simulink model "FlightDataRecorder"  (R2023b)
settings: Solver=VariableStepAuto  StartTime=0.0  StopTime=inf  RelTol=1e-3
libraries: dspindex x28, simulink x4, dspnetwork x4, etargetslib x3, aerolibconvert2 x1
(part 1 of 3)
settings Model: Creator=King  LastModifiedBy=ccInnov
settings SolverCC: AlgebraicLoopSolver=TrustRegion
settings DataIOCC: ReturnWorkspaceOutputs=off
settings OptimizationCC: BlockReduction=off
settings DebuggingCC: UnconnectedInputMsg=warning  UnconnectedOutputMsg=warning  UnconnectedLineMsg=warning  ArithmeticOperatorsInVariantConditions=warning
settings ModelReferenceCC: EnableRefExpFcnMdlSchedulingChecks=on
settings SFSimCC: SimUseLocalCustomCode=off  CustomCodeUndefinedFunction=UseInterfaceOnly
settings RTWCC: RTWUseLocalCustomCode=off
settings CodeAppCC: StateflowObjectComments=on

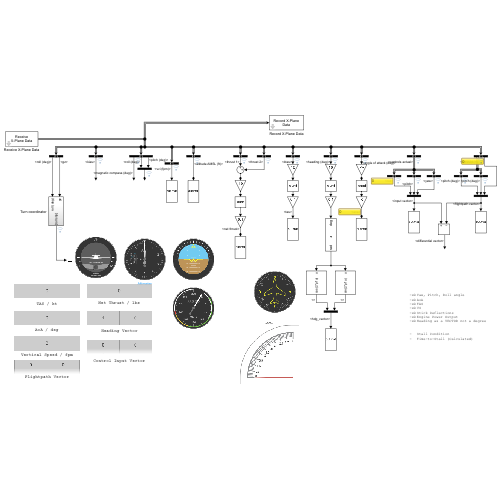
[thumbnail: Simulink's stored preview of the top-level diagram]
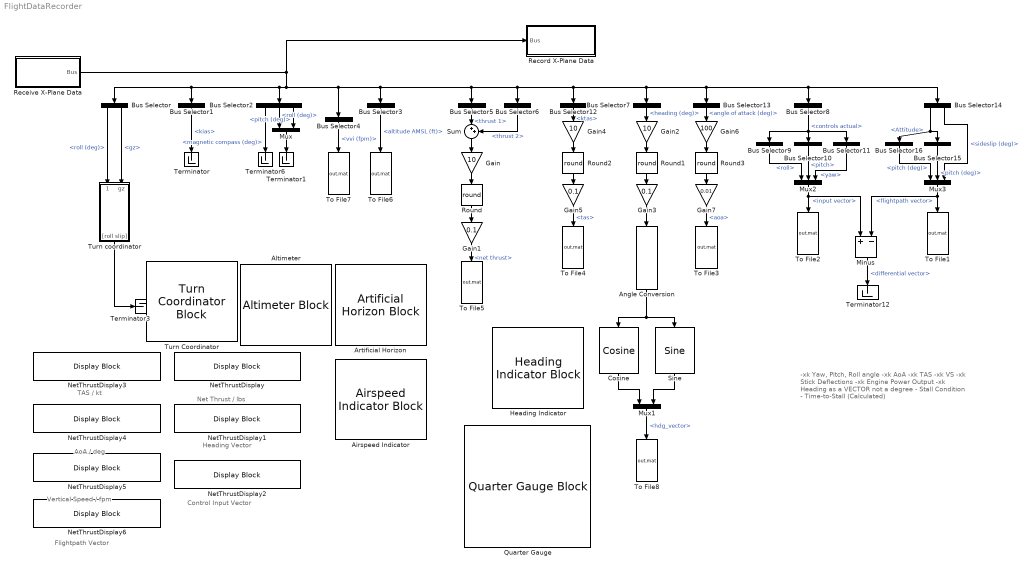
== system FlightDataRecorder ==
  note: -xk Yaw, Pitch, Roll angle
      | -xk AoA
      | -xk TAS
      | -xk VS
      | -xk Stick Deflections
      | -xk Engine Power Output
      | -xk Heading as a VECTOR not a degree
      |
      | - Stall Condition
      | - Time-to-Stall (Calculated)
  note: Net Thrust / lbs
  note: Heading Vector
  note: Control Input Vector
  note: TAS / kt
  note: AoA / deg
  note: Vertical Speed / fpm
  note: Flightpath Vector
  Airspeed Indicator : AirspeedIndicatorBlock  LabelPosition=Hide  ScaleMax=220
  Altimeter : AltimeterBlock  LabelPosition=Hide
  Angle Conversion : aerolibconvert2/Angle Conversion  IU=deg  OU=rad
  Artificial Horizon : ArtificialHorizonBlock  LabelPosition=Hide
  Bus Selector : BusSelector  OutputSignals=AHRS.Attitude.roll (deg),G-loading.gz
  Bus Selector1 : BusSelector  OutputSignals=Speeds.kias
  Bus Selector10 : BusSelector  OutputSignals=pitch
  Bus Selector11 : BusSelector  OutputSignals=yaw
  Bus Selector12 : BusSelector  OutputSignals=Speeds.ktas
  Bus Selector13 : BusSelector  OutputSignals=AHRS.Aerodynamic angles.angle of attack (deg)
  Bus Selector14 : BusSelector  OutputSignals=AHRS.Attitude,AHRS.Aerodynamic angles.sideslip (deg)
  Bus Selector15 : BusSelector  OutputSignals=pitch (deg)
  Bus Selector16 : BusSelector  OutputSignals=pitch (deg)
  Bus Selector2 : BusSelector  OutputSignals=AHRS.Compass.magnetic compass (deg),AHRS.Attitude.roll (deg),AHRS.Attitude.pitch (deg)
  Bus Selector3 : BusSelector  OutputSignals=Location.Geodetic position.altitude AMSL (ft)
  Bus Selector4 : BusSelector  OutputSignals=Speeds.vvi (fpm)
  Bus Selector5 : BusSelector  OutputSignals=Propulsion.Output.Engine thrust (lb).thrust 1
  Bus Selector6 : BusSelector  OutputSignals=Propulsion.Output.Engine thrust (lb).thrust 2
  Bus Selector7 : BusSelector  OutputSignals=AHRS.Attitude.heading (deg)
  Bus Selector8 : BusSelector  OutputSignals=Controls.Controls.controls actual
  Bus Selector9 : BusSelector  OutputSignals=roll
  Cosine : simulink/Lookup Tables/Cosine  Formula=cos(2*pi*u)  NumDataPoints=(2^5)+1  OutputWordLength=16  InternalRulePriority=Speed
  Gain : Gain  Gain=10
  Gain1 : Gain  Gain=0.1
  Gain2 : Gain  Gain=10
  Gain3 : Gain  Gain=0.1
  Gain4 : Gain  Gain=10
  Gain5 : Gain  Gain=0.1
  Gain6 : Gain  Gain=100
  Gain7 : Gain  Gain=0.01
  Heading Indicator : HeadingIndicatorBlock  LabelPosition=Hide
  Minus : Sum  Inputs=+-
  Mux : Mux  Inputs=2
  Mux1 : Mux  Inputs=2
  Mux2 : Mux  Inputs=3
  Mux3 : Mux  Inputs=3
  NetThrustDisplay{,1..6} (7 alike) : DisplayBlock  LabelPosition=Hide  Transparency=1
  Quarter Gauge : QuarterGaugeBlock  ScaleMax=3
  Receive X-Plane Data : Subsystem  mask(Receive X-Plane Data){ipaddress='127.0.0.1', sport=49000, rport=49003, Ts=0.2, p1=on, p2=on, p3=on, p4=off, p12=off, p5=off, p6=on, p7=on, p8=on, p13=off, p10=on, p9=off, p11=off, p16=off, p14=on, p15=off, p17=off, p18=off, p19=off, p20=off}
      mask prompts: ipaddress "X-Plane server IP address:"; sport "X-Plane server port:"; rport "Host data port:"; Ts "Sample time (secs)"; p1 "Time"; p2 "Speeds"; p3 "Main flight controls"; p4 "Other flight controls"; p12 "Cyclics (rotorcraft only)"; p5 "Thrust controls"; p6 "Landing gear"; p7 "AHRS data"; p8 "Engine data"; p13 "Performance data"; p10 "Forces"; p9 "Weights"; p11 "Ground effect"; p16 "Atmospheric data"; p14 "Location"; p15 "Multiplayer position data"; p17 "Power systems"; p18 "Operational systems"; p19 "NAVAID systems"; p20 "Autopilot settings"
      mask help: Configures a running instance of X-Plane to send out selected data and receives a stream of that data over UDP from X-Plane.
      mask Help: Configures a running instance of X-Plane to send out selected data and receives a stream of that data over UDP from X-Plane.
      mask DialogControl ParameterGroupVar Prompt: Network settings
      mask DialogControl Container3 Prompt: Data
      mask Display:
      | disp('Receive\nX-Plane Data')
      | %port_label('output',1,'Bus')
  Record X-Plane Data : Subsystem  mask(Record X-Plane Data){data_name='xpdata'}
      mask prompts: data_name "Data array name:"
      mask help: Records the necessary data from the data bus from the Receive X-Plane Data block for playback with the Send X-Plane Visuals block. The data store is saved to the base workspace as an array, with the X-Plane mission time for indexing the visualisation data as the first row.
      mask Help:
      | Records the necessary data from the data bus from the Receive X-Plane Data block for playback with the Send X-Plane Visuals block. The data store is saved to the base workspace as an array, with the X-Plane mission time for indexing the visualisation data as the first row.
      | 
      | The full set of data saved is:
      | 
      | > Mission time (s)
      | > Latitude (deg)
      | > Longitude (deg)
      | > Altitude MSL (m)
      | > Roll angle (deg)
      | > Pitch angle (deg)
      | > Heading (deg)
      | > Roll stick input
      | > Pitch stick input
      | > Yaw stick input
      | > Flap position
      | > Speedbrake position
      | > Gear deployment
      mask Callback data_name:
      | name = get_param(gcb,'data_name');
      | if ~strcmp(name(1),'''') || ~strcmp(name(end),'''')
      |     error('Could not update data store. Data store name must be specified as a string.',gcb);
      | else
      |     name(1) = []; name(end) = [];
      |     set_param(sprintf('%s/data store',gcb),'VariableName',name);
      | end
      mask Display:
      | disp('Record X-Plane\nData')
      | %port_label('input',1,'bus')
  Round{,1..3} (4 alike) : Rounding  Operator=round
  Sine : simulink/Lookup Tables/Sine  Formula=sin(2*pi*u)  NumDataPoints=(2^5)+1  OutputWordLength=16  InternalRulePriority=Speed
  Sum : Sum  Inputs=|++
  Terminator{,1,3,6,12} (5 alike) : Terminator
  To File1 : ToFile  Filename=out.mat  MatrixName=flightPathVector  SaveFormat=Timeseries
  To File2 : ToFile  Filename=out.mat  MatrixName=inputVector  SaveFormat=Timeseries
  To File3 : ToFile  Filename=out.mat  MatrixName=aoa  SaveFormat=Timeseries
  To File4 : ToFile  Filename=out.mat  MatrixName=tas  SaveFormat=Timeseries
  To File5 : ToFile  Filename=out.mat  MatrixName=netThrust  SaveFormat=Timeseries
  To File6 : ToFile  Filename=out.mat  MatrixName=alt  SaveFormat=Timeseries
  To File7 : ToFile  Filename=out.mat  MatrixName=vertSpeed  SaveFormat=Timeseries
  To File8 : ToFile  Filename=out.mat  MatrixName=headingVector  SaveFormat=Timeseries
  Turn Coordinator : TurnCoordinatorBlock  LabelPosition=Hide
  Turn coordinator : Subsystem
  wires:
  Receive X-Plane Data/1(Bus) -> Record X-Plane Data/1(Bus), Bus Selector/1, Bus Selector1/1, Bus Selector2/1, Bus Selector4/1, Bus Selector12/1, Bus Selector13/1, Bus Selector14/1, Bus Selector8/1, Bus Selector7/1, Bus Selector6/1, Bus Selector5/1, Bus Selector3/1
  Bus Selector1/1 -> Terminator/1  "<kias>"
  Bus Selector2/2 -> Mux/1  "<roll (deg)>"
  Bus Selector2/3 -> Mux/2  "<pitch (deg)>"
  Mux/1 -> Terminator1/1
  Bus Selector3/1 -> To File6/1  "<altitude AMSL (ft)>"
  Bus Selector/1 -> Turn coordinator/1(roll (deg))  "<roll (deg)>"
  Bus Selector/2 -> Turn coordinator/2(gz)  "<gz>"
  Turn coordinator/1("[roll slip]") -> Terminator3/1
  Bus Selector4/1 -> To File7/1  "<vvi (fpm)>"
  Bus Selector2/1 -> Terminator6/1  "<magnetic compass (deg)>"
  Bus Selector5/1 -> Sum/1  "<thrust 1>"
  Bus Selector6/1 -> Sum/2  "<thrust 2>"
  Sum/1 -> Gain/1
  Gain/1 -> Round/1
  Round/1 -> Gain1/1
  Gain1/1 -> To File5/1  "<net thrust>"
  Bus Selector7/1 -> Gain2/1  "<heading (deg)>"
  Gain2/1 -> Round1/1
  Round1/1 -> Gain3/1
  Cosine/1 -> Mux1/1
  Sine/1 -> Mux1/2
  Mux1/1 -> To File8/1  "<hdg_vector>"
  Gain3/1 -> Angle Conversion/1
  Angle Conversion/1 -> Sine/1, Cosine/1
  Bus Selector8/1 -> Bus Selector11/1, Bus Selector10/1, Bus Selector9/1  "<controls actual>"
  Bus Selector10/1 -> Mux2/2  "<pitch>"
  Bus Selector9/1 -> Mux2/1  "<roll>"
  Bus Selector11/1 -> Mux2/3  "<yaw>"
  Mux2/1 -> To File2/1, Minus/1  "<input vector>"
  Gain4/1 -> Round2/1
  Round2/1 -> Gain5/1
  Bus Selector12/1 -> Gain4/1  "<ktas>"
  Gain5/1 -> To File4/1  "<tas>"
  Round3/1 -> Gain7/1
  Gain6/1 -> Round3/1
  Gain7/1 -> To File3/1  "<aoa>"
  Bus Selector13/1 -> Gain6/1  "<angle of attack (deg)>"
  Bus Selector14/1 -> Bus Selector15/1, Bus Selector16/1  "<Attitude>"
  Bus Selector15/1 -> Mux3/2  "<pitch (deg)>"
  Bus Selector16/1 -> Mux3/1  "<pitch (deg)>"
  Bus Selector14/2 -> Mux3/3  "<sideslip (deg)>"
  Mux3/1 -> To File1/1, Minus/2  "<flightpath vector>"
  Minus/1 -> Terminator12/1  "<differential vector>"

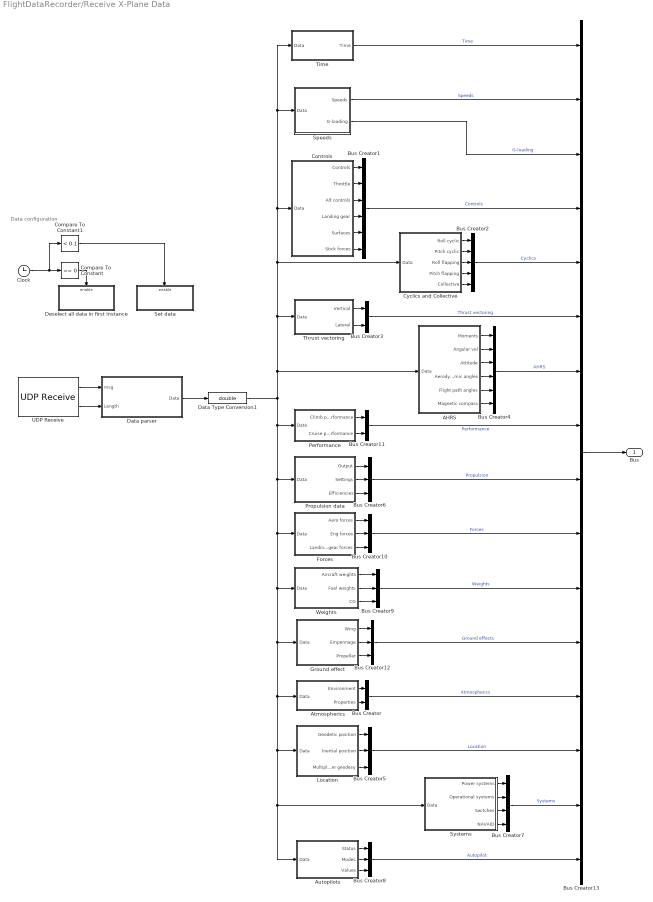
== system FlightDataRecorder/Receive X-Plane Data ==
  note: Data configuration
  AHRS : Subsystem
  Atmospherics : Subsystem
  Autopilots : Subsystem
  Bus Creator : BusCreator  Inputs=2
  Bus Creator1 : BusCreator  Inputs=6
  Bus Creator{5..6,8..10,12} (6 alike) : BusCreator  Inputs=3
  Bus Creator11 : BusCreator  Inputs=2
  Bus Creator13 : BusCreator  Inputs=16
  Bus Creator2 : BusCreator  Inputs=5
  Bus Creator3 : BusCreator  Inputs=2
  Bus Creator4 : BusCreator  Inputs=6
  Bus Creator7 : BusCreator  Inputs=4
  Clock : Clock
  Compare To Constant : simulink/Logic and Bit Operations/Compare To Constant  relop===  const=0  OutDataTypeStr=boolean
  Compare To Constant1 : simulink/Logic and Bit Operations/Compare To Constant  relop=<  const=0.1  OutDataTypeStr=boolean
  Controls : Subsystem
  Cyclics and Collective : Subsystem
  Data Type Conversion1 : DataTypeConversion  OutDataTypeStr=double  SaturateOnIntegerOverflow=off  RndMeth=Floor
  Data parser : MATLAB Function  TreatAsAtomicUnit=on
  Deselect all data in first instance : Subsystem  TreatAsAtomicUnit=on
  Forces : Subsystem
  Ground effect : Subsystem
  Location : Subsystem
  Performance : Subsystem
  Propulsion data : Subsystem
  Set data : Subsystem  TreatAsAtomicUnit=on
  Speeds : Subsystem
  Systems : Subsystem
  Thrust vectoring : Subsystem
  Time : Subsystem
  UDP Receive : dspnetwork/UDP Receive  localURL='0.0.0.0'  localPort=rport  remoteURL=ipaddress  remotePort=-1  recvBufferSize=8794  dims=4397  signalDatatype=uint8  isComplex=off  isVarSize=off  showBlockingTime=on  blockingTime=1  sampletime=Ts  blockPlatform=HOST
  Weights : Subsystem
  Bus : Outport
  wires:
  Controls/5(Surfaces) -> Bus Creator1/5
  Controls/6(Stick forces) -> Bus Creator1/6
  Controls/3(Alt controls) -> Bus Creator1/3
  Thrust vectoring/1(Vertical) -> Bus Creator3/1
  AHRS/6(Magnetic compass) -> Bus Creator4/6
  Controls/4(Landing gear) -> Bus Creator1/4
  AHRS/1(Moments) -> Bus Creator4/1
  Location/1(Geodetic position) -> Bus Creator5/1
  Systems/3(Switches) -> Bus Creator7/3
  Systems/2(Operational systems) -> Bus Creator7/2
  Weights/3(CG) -> Bus Creator9/3
  Location/2(Inertial position) -> Bus Creator5/2
  Cyclics and Collective/4(Pitch flapping) -> Bus Creator2/4
  Cyclics and Collective/2(Pitch cyclic) -> Bus Creator2/2
  Cyclics and Collective/3(Roll flapping) -> Bus Creator2/3
  AHRS/2(Angular vel) -> Bus Creator4/2
  Thrust vectoring/2(Lateral) -> Bus Creator3/2
  AHRS/3(Attitude) -> Bus Creator4/3
  AHRS/4(Aerodynamic angles) -> Bus Creator4/4
  AHRS/5(Flight path angles) -> Bus Creator4/5
  Controls/2(Throttle) -> Bus Creator1/2
  Systems/4(NAVAID) -> Bus Creator7/4
  Autopilots/2(Modes) -> Bus Creator8/2
  Autopilots/3(Values) -> Bus Creator8/3
  Location/3(Multiplayer geodesy) -> Bus Creator5/3
  Autopilots/1(Status) -> Bus Creator8/1
  Controls/1(Controls) -> Bus Creator1/1
  Weights/2(Fuel weights) -> Bus Creator9/2
  Weights/1(Aircraft weights) -> Bus Creator9/1
  Forces/1(Aero forces) -> Bus Creator10/1
  Cyclics and Collective/1(Roll cyclic) -> Bus Creator2/1
  Systems/1(Power systems) -> Bus Creator7/1
  Forces/2(Eng forces) -> Bus Creator10/2
  Forces/3(Landing gear forces) -> Bus Creator10/3
  Propulsion data/1(Output) -> Bus Creator6/1
  Ground effect/2(Empennage) -> Bus Creator12/2
  Time/1(Time) -> Bus Creator13/1  "Time"
  Propulsion data/3(Efficiencies) -> Bus Creator6/3
  Speeds/2(G-loading) -> Bus Creator13/3  "G-loading"
  Ground effect/1(Wing) -> Bus Creator12/1
  Ground effect/3(Propeller) -> Bus Creator12/3
  Propulsion data/2(Settings) -> Bus Creator6/2
  Speeds/1(Speeds) -> Bus Creator13/2  "Speeds"
  Bus Creator13/1 -> Bus/1
  Data Type Conversion1/1 -> Performance/1(Data), Forces/1(Data), Atmospherics/1(Data), Location/1(Data), Autopilots/1(Data), Systems/1(Data), Ground effect/1(Data), Weights/1(Data), Propulsion data/1(Data), AHRS/1(Data), Time/1(Data), Speeds/1(Data), Controls/1(Data), Cyclics and Collective/1(Data), Thrust vectoring/1(Data)
  Compare To Constant1/1 -> Set data/Enable
  Clock/1 -> Compare To Constant1/1, Compare To Constant/1
  Compare To Constant/1 -> Deselect all data in first instance/Enable
  UDP Receive/1 -> Data parser/1(msg)
  Data parser/1(Data) -> Data Type Conversion1/1
  UDP Receive/2 -> Data parser/2(Length)
  Cyclics and Collective/5(Collective) -> Bus Creator2/5
  Performance/1(Climb performance) -> Bus Creator11/1
  Performance/2(Cruise performance) -> Bus Creator11/2
  Atmospherics/2(Properties) -> Bus Creator/2
  Atmospherics/1(Environment) -> Bus Creator/1
  Bus Creator1/1 -> Bus Creator13/4  "Controls"
  Bus Creator2/1 -> Bus Creator13/5  "Cyclics"
  Bus Creator3/1 -> Bus Creator13/6  "Thrust vectoring"
  Bus Creator4/1 -> Bus Creator13/7  "AHRS"
  Bus Creator11/1 -> Bus Creator13/8  "Performance"
  Bus Creator6/1 -> Bus Creator13/9  "Propulsion"
  Bus Creator10/1 -> Bus Creator13/10  "Forces"
  Bus Creator9/1 -> Bus Creator13/11  "Weights"
  Bus Creator12/1 -> Bus Creator13/12  "Ground effects"
  Bus Creator/1 -> Bus Creator13/13  "Atmospherics"
  Bus Creator5/1 -> Bus Creator13/14  "Location"
  Bus Creator7/1 -> Bus Creator13/15  "Systems"
  Bus Creator8/1 -> Bus Creator13/16  "Autopilot"

== system FlightDataRecorder/Record X-Plane Data ==
  Bus : Inport
  Bus Selector : BusSelector  OutputSignals=Time.mission time,Location.Geodetic position.latitude (deg),Location.Geodetic position.longitude (deg),Location.Geodetic position.altitude AMSL (ft),AHRS.Attitude.roll (deg),AHRS.Attitude.pitch (deg),AHRS.Attitude.heading (deg),Controls.Controls.controls actual.roll,Controls.Controls.controls actual.pitch,Controls.Controls.controls actual.yaw,Controls.Controls.trim tabs.flap position,Controls.Controls.trim tabs.speedbrake actual,Controls.Landing gear.gear status  OutputAsBus=on
  data store : ToWorkspace  VariableName=xpdata  SampleTime=-1
      settings: Save2DSignal=2-D array (concatenate along first dimension)
  wires:
  Bus/1 -> Bus Selector/1
  Bus Selector/1 -> data store/1

== system FlightDataRecorder/Turn coordinator ==
  roll (deg) : Inport
  gz : Inport  Port=2
  Bias : Bias  Bias=-1  SaturateOnIntegerOverflow=off
  Gain : Gain  Gain=-1
  Mux4 : Mux  Inputs=2
  Product : Product
  Sign : Signum
  "[roll slip]" : Outport
  wires:
  Mux4/1 -> "[roll slip]"/1
  Sign/1 -> Product/1
  Bias/1 -> Product/2
  Product/1 -> Gain/1
  roll (deg)/1 -> Sign/1, Mux4/1
  gz/1 -> Bias/1
  Gain/1 -> Mux4/2

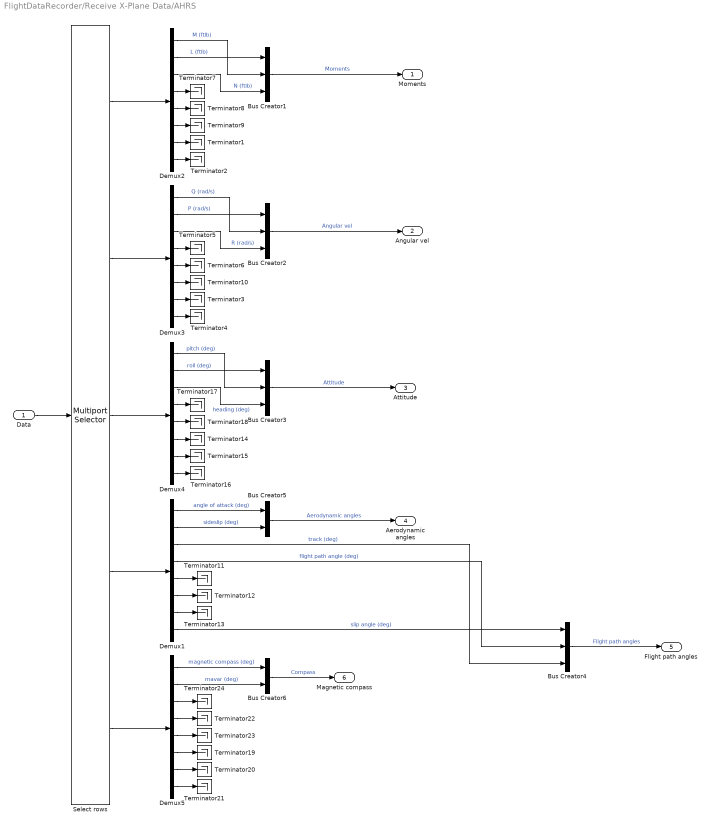
== system FlightDataRecorder/Receive X-Plane Data/AHRS ==
  Data : Inport
  Bus Creator{1..4} (4 alike) : BusCreator  Inputs=3
  Bus Creator5 : BusCreator  Inputs=2
  Bus Creator6 : BusCreator  Inputs=2
  Demux{1..5} (5 alike) : Demux  Outputs=8
  Select rows : dspindex/Multiport Selector  rowsOrCols=Rows  idxCellArray={16,17,18,19,20}  idxErrMode=Clip Index
  Terminator{1..24} (24 alike) : Terminator
  Moments : Outport
  Angular vel : Outport  Port=2
  Attitude : Outport  Port=3
  Aerodynamic angles : Outport  Port=4
  Flight path angles : Outport  Port=5
  Magnetic compass : Outport  Port=6
  wires:
  Bus Creator1/1 -> Moments/1  "Moments"
  Select rows/3 -> Demux4/1
  Select rows/2 -> Demux3/1
  Select rows/1 -> Demux2/1
  Data/1 -> Select rows/1
  Demux2/3 -> Bus Creator1/3  "N (ftlb)"
  Demux2/4 -> Terminator7/1
  Demux2/5 -> Terminator8/1
  Demux2/6 -> Terminator9/1
  Demux2/7 -> Terminator1/1
  Demux2/8 -> Terminator2/1
  Demux3/4 -> Terminator5/1
  Demux3/5 -> Terminator6/1
  Demux3/6 -> Terminator10/1
  Demux3/7 -> Terminator3/1
  Demux3/8 -> Terminator4/1
  Demux3/3 -> Bus Creator2/3  "R (rad/s)"
  Bus Creator2/1 -> Angular vel/1  "Angular vel"
  Demux4/3 -> Bus Creator3/3  "heading (deg)"
  Select rows/4 -> Demux1/1
  Demux1/1 -> Bus Creator5/1  "angle of attack (deg)"
  Demux1/2 -> Bus Creator5/2  "sideslip (deg)"
  Bus Creator3/1 -> Attitude/1  "Attitude"
  Bus Creator5/1 -> Aerodynamic angles/1  "Aerodynamic angles"
  Demux1/4 -> Bus Creator4/2  "flight path angle (deg)"
  Demux1/5 -> Terminator11/1
  Demux1/6 -> Terminator12/1
  Demux1/7 -> Terminator13/1
  Demux4/5 -> Terminator18/1
  Demux4/4 -> Terminator17/1
  Demux4/6 -> Terminator14/1
  Demux4/7 -> Terminator15/1
  Demux4/8 -> Terminator16/1
  Demux5/4 -> Terminator22/1
  Demux5/6 -> Terminator19/1
  Demux5/5 -> Terminator23/1
  Demux5/7 -> Terminator20/1
  Demux5/8 -> Terminator21/1
  Demux5/3 -> Terminator24/1
  Demux5/1 -> Bus Creator6/1  "magnetic compass (deg)"
  Demux5/2 -> Bus Creator6/2  "mavar (deg)"
  Bus Creator4/1 -> Flight path angles/1  "Flight path angles"
  Demux1/8 -> Bus Creator4/1  "slip angle (deg)"
  Demux1/3 -> Bus Creator4/3  "track (deg)"
  Bus Creator6/1 -> Magnetic compass/1  "Compass"
  Select rows/5 -> Demux5/1
  Demux4/1 -> Bus Creator3/2  "pitch (deg)"
  Demux4/2 -> Bus Creator3/1  "roll (deg)"
  Demux2/2 -> Bus Creator1/1  "L (ftlb)"
  Demux2/1 -> Bus Creator1/2  "M (ftlb)"
  Demux3/1 -> Bus Creator2/2  "Q (rad/s)"
  Demux3/2 -> Bus Creator2/1  "P (rad/s)"

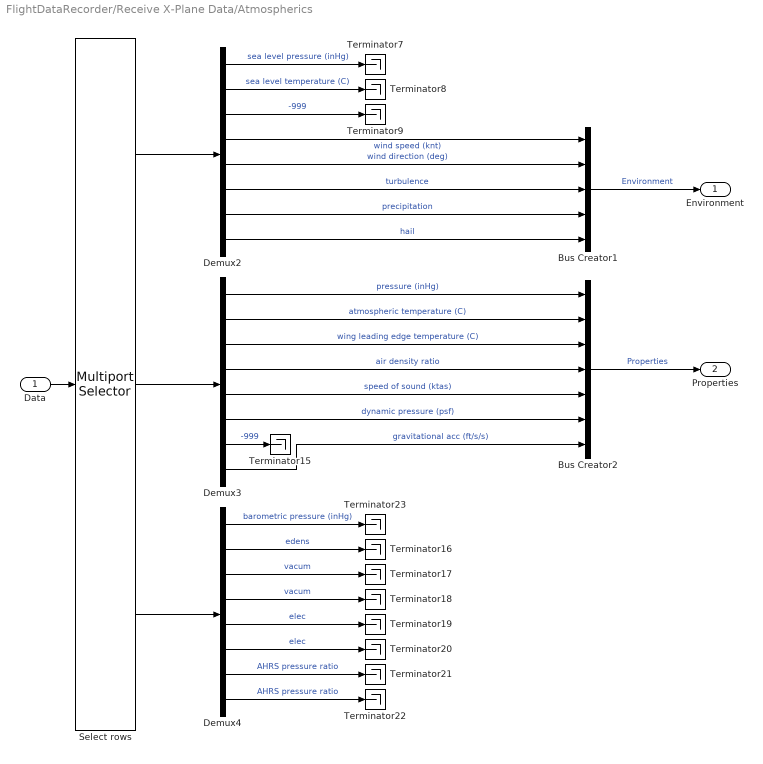
== system FlightDataRecorder/Receive X-Plane Data/Atmospherics ==
  Data : Inport
  Bus Creator1 : BusCreator  Inputs=5
  Bus Creator2 : BusCreator  Inputs=7
  Demux2 : Demux  Outputs=8
  Demux3 : Demux  Outputs=8
  Demux4 : Demux  Outputs=8
  Select rows : dspindex/Multiport Selector  rowsOrCols=Rows  idxCellArray={6,7,8}  idxErrMode=Clip Index
  Terminator{7..9,15..23} (12 alike) : Terminator
  Environment : Outport
  Properties : Outport  Port=2
  wires:
  Data/1 -> Select rows/1
  Select rows/1 -> Demux2/1
  Select rows/2 -> Demux3/1
  Select rows/3 -> Demux4/1
  Demux2/1 -> Terminator7/1  "sea level pressure (inHg)"
  Demux2/2 -> Terminator8/1  "sea level temperature (C)"
  Demux2/3 -> Terminator9/1  "-999"
  Demux3/7 -> Terminator15/1  "-999"
  Demux4/1 -> Terminator23/1  "barometric pressure (inHg)"
  Demux4/2 -> Terminator16/1  "edens"
  Demux4/3 -> Terminator17/1  "vacum"
  Demux4/4 -> Terminator18/1  "vacum"
  Demux4/5 -> Terminator19/1  "elec"
  Demux4/6 -> Terminator20/1  "elec"
  Demux4/7 -> Terminator21/1  "AHRS pressure ratio"
  Demux4/8 -> Terminator22/1  "AHRS pressure ratio"
  Bus Creator2/1 -> Properties/1  "Properties"
  Bus Creator1/1 -> Environment/1  "Environment"
  Demux2/4 -> Bus Creator1/1  "wind speed (knt)"
  Demux2/5 -> Bus Creator1/2  "wind direction (deg)"
  Demux2/6 -> Bus Creator1/3  "turbulence"
  Demux2/7 -> Bus Creator1/4  "precipitation"
  Demux2/8 -> Bus Creator1/5  "hail"
  Demux3/1 -> Bus Creator2/1  "pressure (inHg)"
  Demux3/2 -> Bus Creator2/2  "atmospheric temperature (C)"
  Demux3/3 -> Bus Creator2/3  "wing leading edge temperature (C)"
  Demux3/4 -> Bus Creator2/4  "air density ratio"
  Demux3/5 -> Bus Creator2/5  "speed of sound (ktas)"
  Demux3/6 -> Bus Creator2/6  "dynamic pressure (psf)"
  Demux3/8 -> Bus Creator2/7  "gravitational acc (ft/s/s)"

== system FlightDataRecorder/Receive X-Plane Data/Autopilots ==
  Data : Inport
  Bus Creator10 : BusCreator  Inputs=8
  Bus Creator12 : BusCreator  Inputs=6
  Bus Creator13 : BusCreator  Inputs=8
  Demux11 : Demux  Outputs=8
  Demux12 : Demux  Outputs=8
  Demux13 : Demux  Outputs=8
  Select rows1 : dspindex/Multiport Selector  rowsOrCols=Rows  idxCellArray={117,118,119}  idxErrMode=Clip Index
  Terminator17 : Terminator
  Terminator18 : Terminator
  Status : Outport
  Modes : Outport  Port=2
  Values : Outport  Port=3
  wires:
  Demux13/7 -> Bus Creator13/7  "roll sync"
  Demux13/4 -> Bus Creator13/4  "altitude dial"
  Demux13/6 -> Bus Creator13/6  "altitude use"
  Demux13/8 -> Bus Creator13/8  "pitch sync"
  Demux13/5 -> Bus Creator13/5  "vnav dial"
  Demux13/3 -> Bus Creator13/3  "vvi cmd"
  Demux13/2 -> Bus Creator13/2  "heading cmd"
  Demux13/1 -> Bus Creator13/1  "speed cmd"
  Bus Creator13/1 -> Values/1  "Autopilot values"
  Select rows1/3 -> Demux13/1
  Demux12/7 -> Terminator18/1
  Demux12/8 -> Bus Creator12/6  "sync"
  Demux12/4 -> Terminator17/1
  Demux12/6 -> Bus Creator12/5  "app"
  Demux12/5 -> Bus Creator12/4  "bac"
  Demux12/3 -> Bus Creator12/3  "altitude"
  Demux12/2 -> Bus Creator12/2  "heading"
  Demux12/1 -> Bus Creator12/1  "autothrottle"
  Bus Creator12/1 -> Modes/1  "Autopilot modes"
  Select rows1/2 -> Demux12/1
  Demux11/7 -> Bus Creator10/7  "gp enabled"
  Demux11/4 -> Bus Creator10/4  "vnav enabled"
  Demux11/6 -> Bus Creator10/6  "vnav time"
  Demux11/8 -> Bus Creator10/8  "app type"
  Demux11/5 -> Bus Creator10/5  "vnav armed"
  Demux11/3 -> Bus Creator10/3  "app armed"
  Demux11/2 -> Bus Creator10/2  "alt armed"
  Demux11/1 -> Bus Creator10/1  "nav armed"
  Bus Creator10/1 -> Status/1  "Autopilot arming"
  Select rows1/1 -> Demux11/1
  Data/1 -> Select rows1/1

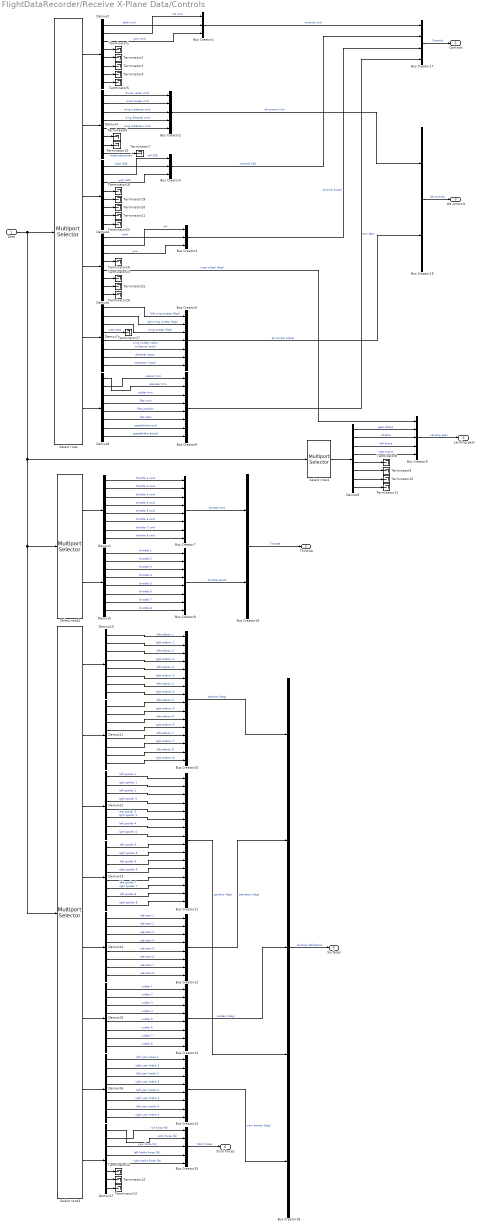
== system FlightDataRecorder/Receive X-Plane Data/Controls ==
  Data : Inport
  Bus Creator1 : BusCreator  Inputs=3
  Bus Creator10 : BusCreator  Inputs=16
  Bus Creator11 : BusCreator  Inputs=16
  Bus Creator{6..8,12..14} (6 alike) : BusCreator  Inputs=8
  Bus Creator{2,9,15,18} (4 alike) : BusCreator  Inputs=5
  Bus Creator16 : BusCreator  Inputs=2
  Bus Creator17 : BusCreator  Inputs=4
  Bus Creator19 : BusCreator  Inputs=2
  Bus Creator3 : BusCreator  Inputs=3
  Bus Creator4 : BusCreator  Inputs=3
  Bus Creator5 : BusCreator  Inputs=7
  Demux{1..17} (17 alike) : Demux  Outputs=8
  Select rows : dspindex/Multiport Selector  rowsOrCols=Rows  idxCellArray={9,10,11,12,13,14}  idxErrMode=Clip Index
  Select rows1 : dspindex/Multiport Selector  rowsOrCols=Rows  idxCellArray={15}  idxErrMode=Clip Index
  Select rows2 : dspindex/Multiport Selector  rowsOrCols=Rows  idxCellArray={26,27}  idxErrMode=Clip Index
  Select rows3 : dspindex/Multiport Selector  rowsOrCols=Rows  idxCellArray={71,72,73,74,75,76,77,78}  idxErrMode=Clip Index
  Terminator{1..23,25..26} (25 alike) : Terminator
  Controls : Outport
  Throttle : Outport  Port=2
  Alt controls : Outport  Port=3
  Landing gear : Outport  Port=4
  Surfaces : Outport  Port=5
  Stick forces : Outport  Port=6
  wires:
  Demux4/8 -> Terminator22/1
  Demux4/7 -> Terminator21/1
  Demux4/6 -> Terminator20/1
  Demux4/5 -> Terminator19/1
  Demux4/4 -> Terminator18/1
  Demux4/3 -> Bus Creator3/3  "yaw SAS"
  Demux3/7 -> Terminator15/1
  Select rows/3 -> Demux4/1
  Select rows/2 -> Demux3/1
  Select rows/1 -> Demux2/1
  Data/1 -> Select rows3/1, Select rows2/1, Select rows1/1, Select rows/1
  Demux2/4 -> Terminator1/1
  Demux2/5 -> Terminator2/1
  Demux2/6 -> Terminator3/1
  Demux2/7 -> Terminator4/1
  Demux2/8 -> Terminator5/1
  Demux2/3 -> Bus Creator1/3  "yaw cmd"
  Demux3/1 -> Bus Creator2/1  "thrust vector cmd"
  Demux3/2 -> Bus Creator2/2  "wind sweep cmd"
  Demux3/3 -> Bus Creator2/3  "wing incidence cmd"
  Demux3/4 -> Bus Creator2/4  "wing dihedral cmd"
  Demux3/5 -> Bus Creator2/5  "wing retraction cmd"
  Demux3/8 -> Terminator7/1  "water jettisoned"
  Demux3/6 -> Terminator6/1
  Select rows2/2 -> Demux5/1
  Select rows2/1 -> Demux1/1
  Bus Creator3/1 -> Bus Creator17/2  "controls SAS"
  Demux6/8 -> Terminator26/1
  Demux6/7 -> Terminator25/1
  Demux6/6 -> Terminator23/1
  Demux6/5 -> Bus Creator9/1  "nose wheel (deg)"
  Demux6/4 -> Terminator16/1
  Demux6/3 -> Bus Creator4/3  "yaw"
  Select rows/4 -> Demux6/1
  Select rows/5 -> Demux7/1
  Demux7/1 -> Bus Creator5/1  "left wing sweep (deg)"
  Demux7/3 -> Bus Creator5/3  "wing sweep (deg)"
  Demux7/4 -> Terminator17/1  "vect ratio"
  Demux7/5 -> Bus Creator5/4  "wing sweep (ratio)"
  Demux7/6 -> Bus Creator5/5  "incidence (ratio)"
  Demux7/7 -> Bus Creator5/6  "dihedral (ratio)"
  Demux7/8 -> Bus Creator5/7  "retraction (ratio)"
  Demux7/2 -> Bus Creator5/2  "right wing sweep (deg)"
  Select rows/6 -> Demux8/1
  Demux8/3 -> Bus Creator6/3  "rudder trim"
  Demux8/4 -> Bus Creator6/4  "flap cmd"
  Demux8/7 -> Bus Creator6/7  "speedbrake cmd"
  Demux8/5 -> Bus Creator6/5  "flap position"
  Demux8/6 -> Bus Creator6/6  "slat ratio"
  Demux8/8 -> Bus Creator6/8  "speedbrake actual"
  Bus Creator6/1 -> Bus Creator17/4  "trim tabs"
  Demux1/3 -> Bus Creator7/3  "throttle 3 cmd"
  Demux1/4 -> Bus Creator7/4  "throttle 4 cmd"
  Demux1/2 -> Bus Creator7/2  "throttle 2 cmd"
  Demux1/1 -> Bus Creator7/1  "throttle 1 cmd"
  Demux1/8 -> Bus Creator7/8  "throttle 8 cmd"
  Demux1/7 -> Bus Creator7/7  "throttle 7 cmd"
  Demux1/5 -> Bus Creator7/5  "throttle 5 cmd"
  Demux1/6 -> Bus Creator7/6  "throttle 6 cmd"
  Demux5/3 -> Bus Creator8/3  "throttle 3"
  Demux5/6 -> Bus Creator8/6  "throttle 6"
  Demux5/8 -> Bus Creator8/8  "throttle 8"
  Demux5/2 -> Bus Creator8/2  "throttle 2"
  Demux5/4 -> Bus Creator8/4  "throttle 4"
  Demux5/1 -> Bus Creator8/1  "throttle 1"
  Demux5/7 -> Bus Creator8/7  "throttle 7"
  Demux5/5 -> Bus Creator8/5  "throttle 5"
  Bus Creator8/1 -> Bus Creator16/2  "throttle actual"
  Bus Creator4/1 -> Bus Creator17/3  "controls actual"
  Bus Creator2/1 -> Bus Creator19/1  "alt control cmd"
  Select rows1/1 -> Demux9/1
  Demux9/5 -> Terminator8/1
  Demux9/6 -> Terminator9/1
  Demux9/7 -> Terminator10/1
  Demux9/8 -> Terminator11/1
  Demux9/1 -> Bus Creator9/2  "gear status"
  Demux9/2 -> Bus Creator9/3  "wbrake"
  Demux9/3 -> Bus Creator9/4  "left brake"
  Demux9/4 -> Bus Creator9/5  "right brake"
  Bus Creator9/1 -> Landing gear/1  "Landing gear"
  Demux10/3 -> Bus Creator10/3  "left aileron 2"
  Demux10/6 -> Bus Creator10/6  "right aileron 3"
  Demux10/8 -> Bus Creator10/8  "right aileron 4"
  Demux10/2 -> Bus Creator10/2  "right aileron 1"
  Demux10/4 -> Bus Creator10/4  "right aileron 2"
  Demux10/7 -> Bus Creator10/7  "left aileron 4"
  Demux10/5 -> Bus Creator10/5  "left aileron 3"
  Bus Creator10/1 -> Bus Creator18/1  "ailerons (deg)"
  Select rows3/1 -> Demux10/1
  Demux10/1 -> Bus Creator10/1  "left aileron 1"
  Demux11/3 -> Bus Creator10/11  "left aileron 6"
  Demux11/6 -> Bus Creator10/14  "right aileron 7"
  Demux11/8 -> Bus Creator10/16  "right aileron 8"
  Demux11/2 -> Bus Creator10/10  "right aileron 5"
  Demux11/4 -> Bus Creator10/12  "right aileron 6"
  Demux11/7 -> Bus Creator10/15  "left aileron 8"
  Demux11/5 -> Bus Creator10/13  "left aileron 7"
  Select rows3/2 -> Demux11/1
  Demux11/1 -> Bus Creator10/9  "left aileron 5"
  Demux12/3 -> Bus Creator11/3  "left spoiler 2"
  Demux12/6 -> Bus Creator11/6  "right spoiler 3"
  Demux12/8 -> Bus Creator11/8  "right spoiler 4"
  Demux12/2 -> Bus Creator11/2  "right spoiler 1"
  Demux12/4 -> Bus Creator11/4  "right spoiler 2"
  Demux12/7 -> Bus Creator11/7  "left spoiler 4"
  Demux12/5 -> Bus Creator11/5  "left spoiler 3"
  Select rows3/3 -> Demux12/1
  Demux12/1 -> Bus Creator11/1  "left spoiler 1"
  Demux13/3 -> Bus Creator11/11  "left spoiler 6"
  Demux13/6 -> Bus Creator11/14  "right spoiler 7"
  Demux13/8 -> Bus Creator11/16  "right spoiler 8"
  Demux13/2 -> Bus Creator11/10  "right spoiler 5"
  Demux13/4 -> Bus Creator11/12  "right spoiler 6"
  Demux13/7 -> Bus Creator11/15  "left spoiler 8"
  Demux13/5 -> Bus Creator11/13  "left spoiler 7"
  Select rows3/4 -> Demux13/1
  Demux13/1 -> Bus Creator11/9  "left spoiler 5"
  Select rows3/5 -> Demux14/1
  Demux14/3 -> Bus Creator12/3  "elevator 3"
  Demux14/6 -> Bus Creator12/6  "elevator 6"
  Demux14/8 -> Bus Creator12/8  "elevator 8"
  Demux14/2 -> Bus Creator12/2  "elevator 2"
  Demux14/4 -> Bus Creator12/4  "elevator 4"
  Demux14/1 -> Bus Creator12/1  "elevator 1"
  Demux14/7 -> Bus Creator12/7  "elevator 7"
  Demux14/5 -> Bus Creator12/5  "elevator 5"
  Select rows3/6 -> Demux15/1
  Demux15/3 -> Bus Creator13/3  "rudder 3"
  Demux15/6 -> Bus Creator13/6  "rudder 6"
  Demux15/8 -> Bus Creator13/8  "rudder 8"
  Demux15/2 -> Bus Creator13/2  "rudder 2"
  Demux15/4 -> Bus Creator13/4  "rudder 4"
  Demux15/1 -> Bus Creator13/1  "rudder 1"
  Demux15/7 -> Bus Creator13/7  "rudder 7"
  Demux15/5 -> Bus Creator13/5  "rudder 5"
  Select rows3/7 -> Demux16/1
  Demux16/3 -> Bus Creator14/3  "left yaw brake 2"
  Demux16/6 -> Bus Creator14/6  "right yaw brake 3"
  Demux16/8 -> Bus Creator14/8  "right yaw brake 4"
  Demux16/2 -> Bus Creator14/2  "right yaw brake 1"
  Demux16/4 -> Bus Creator14/4  "right yaw brake 2"
  Demux16/1 -> Bus Creator14/1  "left yaw brake 1"
  Demux16/7 -> Bus Creator14/7  "left yaw brake 4"
  Demux16/5 -> Bus Creator14/5  "left yaw brake 3"
  Select rows3/8 -> Demux17/1
  Demux17/3 -> Bus Creator15/3  "yaw force (lb)"
  Demux17/4 -> Bus Creator15/4  "left brake force (lb)"
  Demux17/5 -> Bus Creator15/5  "right brake force (lb)"
  Demux17/7 -> Terminator12/1
  Demux17/8 -> Terminator13/1
  Demux17/6 -> Terminator14/1
  Bus Creator7/1 -> Bus Creator16/1  "throttle cmd"
  Bus Creator16/1 -> Throttle/1  "Throttle"
  Bus Creator1/1 -> Bus Creator17/1  "controls cmd"
  Bus Creator17/1 -> Controls/1  "Controls"
  Bus Creator14/1 -> Bus Creator18/5  "yaw brakes (deg)"
  Bus Creator18/1 -> Surfaces/1  "Surface deflections"
  Bus Creator15/1 -> Stick forces/1  "Stick forces"
  Bus Creator5/1 -> Bus Creator19/2  "alt control actual"
  Bus Creator19/1 -> Alt controls/1  "Alt controls"
  Demux2/2 -> Bus Creator1/1  "roll cmd"
  Demux2/1 -> Bus Creator1/2  "pitch cmd"
  Demux4/2 -> Bus Creator3/1  "roll SAS"
  Demux4/1 -> Bus Creator3/2  "pitch SAS"
  Demux6/2 -> Bus Creator4/1  "roll"
  Demux6/1 -> Bus Creator4/2  "pitch"
  Demux8/2 -> Bus Creator6/1  "aileron trim"
  Demux8/1 -> Bus Creator6/2  "elevator trim"
  Demux17/2 -> Bus Creator15/1  "roll force (lb)"
  Demux17/1 -> Bus Creator15/2  "pitch force (lb)"
  Bus Creator12/1 -> Bus Creator18/2  "elevators (deg)"
  Bus Creator13/1 -> Bus Creator18/3  "rudders (deg)"
  Bus Creator11/1 -> Bus Creator18/4  "spoilers (deg)"

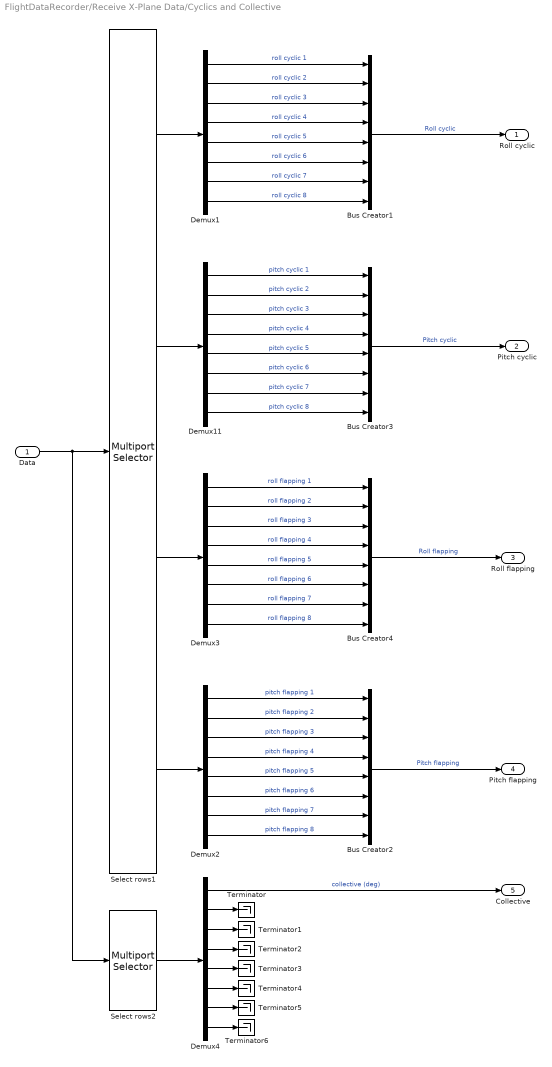
== system FlightDataRecorder/Receive X-Plane Data/Cyclics and Collective ==
  Data : Inport
  Bus Creator{1..4} (4 alike) : BusCreator  Inputs=8
  Demux{1..4,11} (5 alike) : Demux  Outputs=8
  Select rows1 : dspindex/Multiport Selector  rowsOrCols=Rows  idxCellArray={82,81,84,83}  idxErrMode=Clip Index
  Select rows2 : dspindex/Multiport Selector  rowsOrCols=Rows  idxCellArray={40}  idxErrMode=Clip Index
  Terminator{,1..6} (7 alike) : Terminator
  Roll cyclic : Outport
  Pitch cyclic : Outport  Port=2
  Roll flapping : Outport  Port=3
  Pitch flapping : Outport  Port=4
  Collective : Outport  Port=5
  wires:
  Data/1 -> Select rows2/1, Select rows1/1
  Demux11/4 -> Bus Creator3/4  "pitch cyclic 4"
  Demux11/3 -> Bus Creator3/3  "pitch cyclic 3"
  Demux11/2 -> Bus Creator3/2  "pitch cyclic 2"
  Demux11/1 -> Bus Creator3/1  "pitch cyclic 1"
  Demux11/5 -> Bus Creator3/5  "pitch cyclic 5"
  Demux11/6 -> Bus Creator3/6  "pitch cyclic 6"
  Demux11/8 -> Bus Creator3/8  "pitch cyclic 8"
  Demux11/7 -> Bus Creator3/7  "pitch cyclic 7"
  Demux1/4 -> Bus Creator1/4  "roll cyclic 4"
  Demux1/3 -> Bus Creator1/3  "roll cyclic 3"
  Demux1/2 -> Bus Creator1/2  "roll cyclic 2"
  Demux1/1 -> Bus Creator1/1  "roll cyclic 1"
  Demux1/5 -> Bus Creator1/5  "roll cyclic 5"
  Demux1/6 -> Bus Creator1/6  "roll cyclic 6"
  Demux1/8 -> Bus Creator1/8  "roll cyclic 8"
  Demux1/7 -> Bus Creator1/7  "roll cyclic 7"
  Demux2/4 -> Bus Creator2/4  "pitch flapping 4"
  Demux2/3 -> Bus Creator2/3  "pitch flapping 3"
  Demux2/2 -> Bus Creator2/2  "pitch flapping 2"
  Demux2/1 -> Bus Creator2/1  "pitch flapping 1"
  Demux2/5 -> Bus Creator2/5  "pitch flapping 5"
  Demux2/6 -> Bus Creator2/6  "pitch flapping 6"
  Demux2/8 -> Bus Creator2/8  "pitch flapping 8"
  Demux2/7 -> Bus Creator2/7  "pitch flapping 7"
  Demux3/4 -> Bus Creator4/4  "roll flapping 4"
  Demux3/3 -> Bus Creator4/3  "roll flapping 3"
  Demux3/2 -> Bus Creator4/2  "roll flapping 2"
  Demux3/1 -> Bus Creator4/1  "roll flapping 1"
  Demux3/5 -> Bus Creator4/5  "roll flapping 5"
  Demux3/6 -> Bus Creator4/6  "roll flapping 6"
  Demux3/8 -> Bus Creator4/8  "roll flapping 8"
  Demux3/7 -> Bus Creator4/7  "roll flapping 7"
  Select rows1/1 -> Demux1/1
  Bus Creator1/1 -> Roll cyclic/1  "Roll cyclic"
  Select rows1/2 -> Demux11/1
  Bus Creator3/1 -> Pitch cyclic/1  "Pitch cyclic"
  Select rows1/3 -> Demux3/1
  Bus Creator4/1 -> Roll flapping/1  "Roll flapping"
  Select rows1/4 -> Demux2/1
  Bus Creator2/1 -> Pitch flapping/1  "Pitch flapping"
  Select rows2/1 -> Demux4/1
  Demux4/2 -> Terminator/1
  Demux4/8 -> Terminator6/1
  Demux4/7 -> Terminator5/1
  Demux4/6 -> Terminator4/1
  Demux4/5 -> Terminator3/1
  Demux4/4 -> Terminator2/1
  Demux4/3 -> Terminator1/1
  Demux4/1 -> Collective/1  "collective (deg)"

== system FlightDataRecorder/Receive X-Plane Data/Deselect all data in first instance ==
  Enable : EnablePort
  Byte Pack1 : etargetslib/Byte Pack  datatypes={'uint8','uint32'}  byteAlign=1
  UDP Send : dspnetwork/UDP Send  remoteURL=ipaddress  remotePort=sport  localURL='0.0.0.0'  localPortSource=Automatically determine  localPort=-1  sendBufferSize=8192  sampletime=-1  blockPlatform=[]  separateLengthPort=0
  Unselect all data : MATLAB Function  TreatAsAtomicUnit=on
  wires:
  Unselect all data/2(y2) -> Byte Pack1/2
  Byte Pack1/1 -> UDP Send/1
  Unselect all data/1(y1) -> Byte Pack1/1

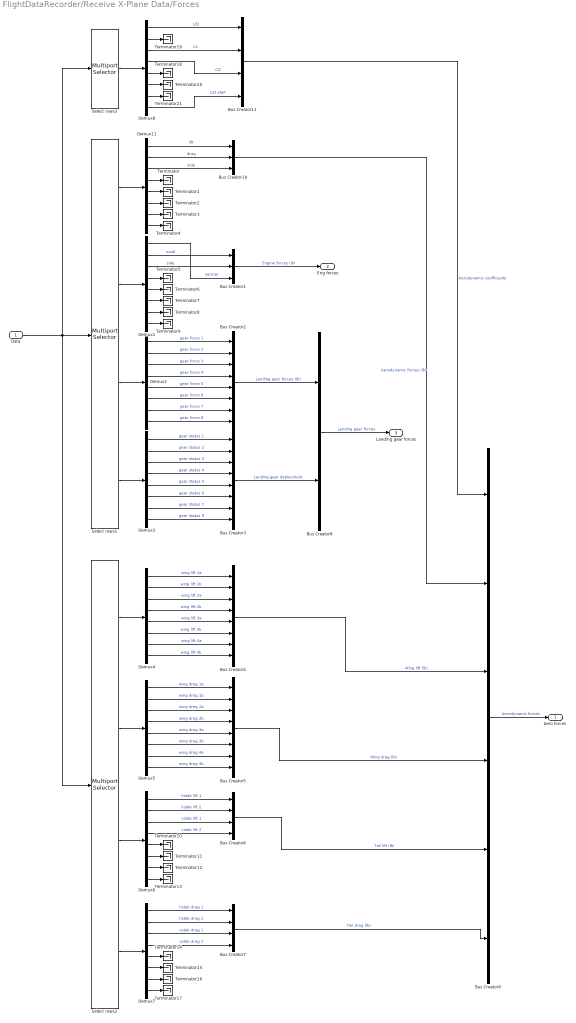
== system FlightDataRecorder/Receive X-Plane Data/Forces ==
  Data : Inport
  Bus Creator1 : BusCreator  Inputs=3
  Bus Creator10 : BusCreator  Inputs=3
  Bus Creator11 : BusCreator  Inputs=4
  Bus Creator{2..5} (4 alike) : BusCreator  Inputs=8
  Bus Creator6 : BusCreator  Inputs=4
  Bus Creator7 : BusCreator  Inputs=4
  Bus Creator8 : BusCreator  Inputs=2
  Bus Creator9 : BusCreator  Inputs=6
  Demux{1..8,11} (9 alike) : Demux  Outputs=8
  Select rows1 : dspindex/Multiport Selector  rowsOrCols=Rows  idxCellArray={65,66,67,68}  idxErrMode=Clip Index
  Select rows2 : dspindex/Multiport Selector  rowsOrCols=Rows  idxCellArray={93,94,95,96}  idxErrMode=Clip Index
  Select rows3 : dspindex/Multiport Selector  rowsOrCols=Rows  idxCellArray={69}  idxErrMode=Clip Index
  Terminator{,1..21} (22 alike) : Terminator
  Aero forces : Outport
  Eng forces : Outport  Port=2
  Landing gear forces : Outport  Port=3
  wires:
  Demux11/3 -> Bus Creator10/3  "side"
  Demux11/2 -> Bus Creator10/2  "drag"
  Demux11/1 -> Bus Creator10/1  "lift"
  Select rows1/1 -> Demux11/1
  Data/1 -> Select rows3/1, Select rows2/1, Select rows1/1
  Demux11/4 -> Terminator/1
  Demux11/8 -> Terminator4/1
  Demux11/7 -> Terminator3/1
  Demux11/6 -> Terminator2/1
  Demux11/5 -> Terminator1/1
  Select rows1/2 -> Demux1/1
  Demux1/4 -> Terminator5/1
  Demux1/8 -> Terminator9/1
  Demux1/7 -> Terminator8/1
  Demux1/6 -> Terminator7/1
  Demux1/5 -> Terminator6/1
  Bus Creator1/1 -> Eng forces/1  "Engine forces (lb)"
  Demux1/1 -> Bus Creator1/3  "normal"
  Demux1/2 -> Bus Creator1/1  "axial"
  Demux1/3 -> Bus Creator1/2  "side"
  Demux2/3 -> Bus Creator2/3  "gear force 3"
  Demux2/2 -> Bus Creator2/2  "gear force 2"
  Demux2/1 -> Bus Creator2/1  "gear force 1"
  Select rows1/3 -> Demux2/1
  Bus Creator2/1 -> Bus Creator8/1  "Landing gear forces (lb)"
  Demux2/7 -> Bus Creator2/7  "gear force 7"
  Demux2/5 -> Bus Creator2/5  "gear force 5"
  Demux2/8 -> Bus Creator2/8  "gear force 8"
  Demux2/6 -> Bus Creator2/6  "gear force 6"
  Demux2/4 -> Bus Creator2/4  "gear force 4"
  Demux3/3 -> Bus Creator3/3  "gear status 3"
  Demux3/2 -> Bus Creator3/2  "gear status 2"
  Demux3/1 -> Bus Creator3/1  "gear status 1"
  Select rows1/4 -> Demux3/1
  Bus Creator3/1 -> Bus Creator8/2  "Landing gear deployment"
  Demux3/7 -> Bus Creator3/7  "gear status 7"
  Demux3/5 -> Bus Creator3/5  "gear status 5"
  Demux3/8 -> Bus Creator3/8  "gear status 8"
  Demux3/6 -> Bus Creator3/6  "gear status 6"
  Demux3/4 -> Bus Creator3/4  "gear status 4"
  Bus Creator8/1 -> Landing gear forces/1  "Landing gear forces"
  Demux4/3 -> Bus Creator4/3  "wing lift 2a"
  Demux4/2 -> Bus Creator4/2  "wing lift 1b"
  Demux4/1 -> Bus Creator4/1  "wing lift 1a"
  Select rows2/1 -> Demux4/1
  Bus Creator4/1 -> Bus Creator9/3  "Wing lift (lb)"
  Demux4/7 -> Bus Creator4/7  "wing lift 4a"
  Demux4/5 -> Bus Creator4/5  "wing lift 3a"
  Demux4/8 -> Bus Creator4/8  "wing lift 4b"
  Demux4/6 -> Bus Creator4/6  "wing lift 3b"
  Demux4/4 -> Bus Creator4/4  "wing lift 2b"
  Demux5/3 -> Bus Creator5/3  "wing drag 2a"
  Demux5/2 -> Bus Creator5/2  "wing drag 1b"
  Demux5/1 -> Bus Creator5/1  "wing drag 1a"
  Select rows2/2 -> Demux5/1
  Bus Creator5/1 -> Bus Creator9/4  "Wing drag (lb)"
  Demux5/7 -> Bus Creator5/7  "wing drag 4a"
  Demux5/5 -> Bus Creator5/5  "wing drag 3a"
  Demux5/8 -> Bus Creator5/8  "wing drag 4b"
  Demux5/6 -> Bus Creator5/6  "wing drag 3b"
  Demux5/4 -> Bus Creator5/4  "wing drag 2b"
  Demux6/3 -> Bus Creator6/3  "vstab lift 1"
  Demux6/2 -> Bus Creator6/2  "hstab lift 2"
  Demux6/1 -> Bus Creator6/1  "hstab lift 1"
  Select rows2/3 -> Demux6/1
  Bus Creator6/1 -> Bus Creator9/5  "Tail lift (lb)"
  Demux6/4 -> Bus Creator6/4  "vstab lift 2"
  Demux6/5 -> Terminator10/1
  Demux6/8 -> Terminator13/1
  Demux6/7 -> Terminator12/1
  Demux6/6 -> Terminator11/1
  Demux7/3 -> Bus Creator7/3  "vstab drag 1"
  Demux7/2 -> Bus Creator7/2  "hstab drag 2"
  Demux7/1 -> Bus Creator7/1  "hstab drag 1"
  Select rows2/4 -> Demux7/1
  Bus Creator7/1 -> Bus Creator9/6  "Tail drag (lb)"
  Demux7/4 -> Bus Creator7/4  "vstab drag 2"
  Demux7/5 -> Terminator14/1
  Demux7/8 -> Terminator17/1
  Demux7/7 -> Terminator16/1
  Demux7/6 -> Terminator15/1
  Bus Creator9/1 -> Aero forces/1  "Aerodynamic forces"
  Bus Creator10/1 -> Bus Creator9/2  "Aerodynamic forces (lb)"
  Demux8/5 -> Terminator18/1
  Demux8/6 -> Terminator20/1
  Demux8/7 -> Terminator21/1
  Select rows3/1 -> Demux8/1
  Demux8/2 -> Terminator19/1
  Demux8/1 -> Bus Creator11/1  "L/D"
  Demux8/3 -> Bus Creator11/2  "CL"
  Demux8/4 -> Bus Creator11/3  "CD"
  Demux8/8 -> Bus Creator11/4  "L/D etaP"
  Bus Creator11/1 -> Bus Creator9/1  "Aerodynamic coefficients"

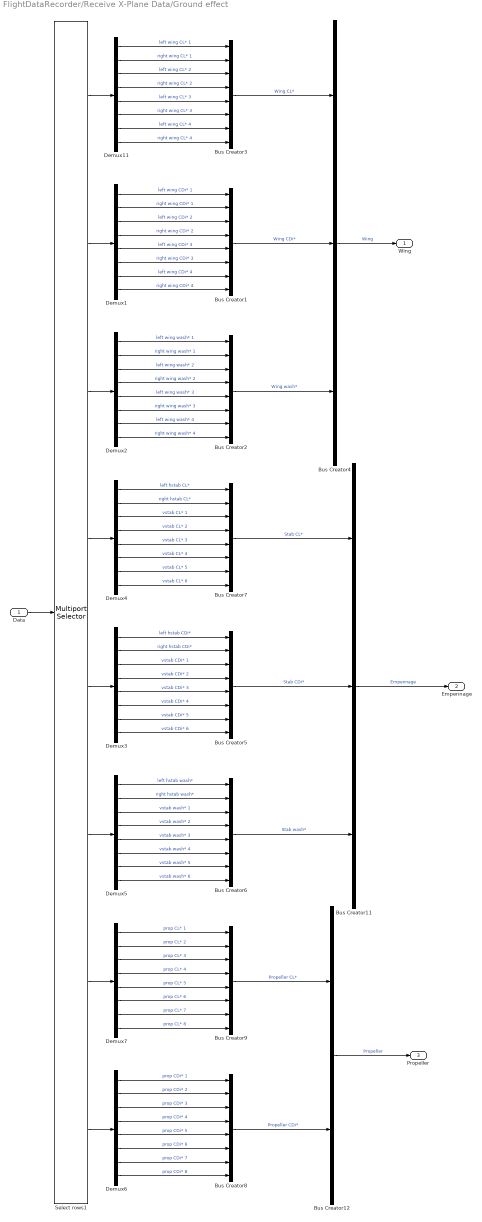
== system FlightDataRecorder/Receive X-Plane Data/Ground effect ==
  Data : Inport
  Bus Creator{1..3,5..9} (8 alike) : BusCreator  Inputs=8
  Bus Creator11 : BusCreator  Inputs=3
  Bus Creator12 : BusCreator  Inputs=2
  Bus Creator4 : BusCreator  Inputs=3
  Demux{1..7,11} (8 alike) : Demux  Outputs=8
  Select rows1 : dspindex/Multiport Selector  rowsOrCols=Rows  idxCellArray={85,86,87,88,89,90,91,92}  idxErrMode=Clip Index
  Wing : Outport
  Empennage : Outport  Port=2
  Propeller : Outport  Port=3
  wires:
  Bus Creator1/1 -> Bus Creator4/2  "Wing CDi*"
  Demux11/7 -> Bus Creator3/7  "left wing CL* 4"
  Demux11/8 -> Bus Creator3/8  "right wing CL* 4"
  Demux11/6 -> Bus Creator3/6  "right wing CL* 3"
  Demux11/5 -> Bus Creator3/5  "left wing CL* 3"
  Demux11/1 -> Bus Creator3/1  "left wing CL* 1"
  Demux11/2 -> Bus Creator3/2  "right wing CL* 1"
  Demux11/3 -> Bus Creator3/3  "left wing CL* 2"
  Demux11/4 -> Bus Creator3/4  "right wing CL* 2"
  Data/1 -> Select rows1/1
  Select rows1/1 -> Demux11/1
  Bus Creator3/1 -> Bus Creator4/1  "Wing CL*"
  Select rows1/2 -> Demux1/1
  Demux1/7 -> Bus Creator1/7  "left wing CDi* 4"
  Demux1/8 -> Bus Creator1/8  "right wing CDi* 4"
  Demux1/6 -> Bus Creator1/6  "right wing CDi* 3"
  Demux1/5 -> Bus Creator1/5  "left wing CDi* 3"
  Demux1/1 -> Bus Creator1/1  "left wing CDi* 1"
  Demux1/2 -> Bus Creator1/2  "right wing CDi* 1"
  Demux1/3 -> Bus Creator1/3  "left wing CDi* 2"
  Demux1/4 -> Bus Creator1/4  "right wing CDi* 2"
  Bus Creator2/1 -> Bus Creator4/3  "Wing wash*"
  Demux2/7 -> Bus Creator2/7  "left wing wash* 4"
  Demux2/8 -> Bus Creator2/8  "right wing wash* 4"
  Demux2/6 -> Bus Creator2/6  "right wing wash* 3"
  Demux2/5 -> Bus Creator2/5  "left wing wash* 3"
  Demux2/1 -> Bus Creator2/1  "left wing wash* 1"
  Demux2/2 -> Bus Creator2/2  "right wing wash* 1"
  Demux2/3 -> Bus Creator2/3  "left wing wash* 2"
  Demux2/4 -> Bus Creator2/4  "right wing wash* 2"
  Select rows1/3 -> Demux2/1
  Bus Creator4/1 -> Wing/1  "Wing"
  Bus Creator5/1 -> Bus Creator11/2  "Stab CDi*"
  Demux4/7 -> Bus Creator7/7  "vstab CL* 5"
  Demux4/8 -> Bus Creator7/8  "vstab CL* 6"
  Demux4/6 -> Bus Creator7/6  "vstab CL* 4"
  Demux4/5 -> Bus Creator7/5  "vstab CL* 3"
  Demux4/1 -> Bus Creator7/1  "left hstab CL*"
  Demux4/2 -> Bus Creator7/2  "right hstab CL*"
  Demux4/3 -> Bus Creator7/3  "vstab CL* 1"
  Demux4/4 -> Bus Creator7/4  "vstab CL* 2"
  Select rows1/4 -> Demux4/1
  Bus Creator7/1 -> Bus Creator11/1  "Stab CL*"
  Select rows1/5 -> Demux3/1
  Demux3/7 -> Bus Creator5/7  "vstab CDi* 5"
  Demux3/8 -> Bus Creator5/8  "vstab CDi* 6"
  Demux3/6 -> Bus Creator5/6  "vstab CDi* 4"
  Demux3/5 -> Bus Creator5/5  "vstab CDi* 3"
  Demux3/1 -> Bus Creator5/1  "left hstab CDi*"
  Demux3/2 -> Bus Creator5/2  "right hstab CDi*"
  Demux3/3 -> Bus Creator5/3  "vstab CDi* 1"
  Demux3/4 -> Bus Creator5/4  "vstab CDi* 2"
  Bus Creator6/1 -> Bus Creator11/3  "Stab wash*"
  Demux5/7 -> Bus Creator6/7  "vstab wash* 5"
  Demux5/8 -> Bus Creator6/8  "vstab wash* 6"
  Demux5/6 -> Bus Creator6/6  "vstab wash* 4"
  Demux5/5 -> Bus Creator6/5  "vstab wash* 3"
  Demux5/1 -> Bus Creator6/1  "left hstab wash*"
  Demux5/2 -> Bus Creator6/2  "right hstab wash*"
  Demux5/3 -> Bus Creator6/3  "vstab wash* 1"
  Demux5/4 -> Bus Creator6/4  "vstab wash* 2"
  Select rows1/6 -> Demux5/1
  Bus Creator8/1 -> Bus Creator12/2  "Propeller CDi*"
  Demux7/7 -> Bus Creator9/7  "prop CL* 7"
  Demux7/8 -> Bus Creator9/8  "prop CL* 8"
  Demux7/6 -> Bus Creator9/6  "prop CL* 6"
  Demux7/5 -> Bus Creator9/5  "prop CL* 5"
  Demux7/1 -> Bus Creator9/1  "prop CL* 1"
  Demux7/2 -> Bus Creator9/2  "prop CL* 2"
  Demux7/3 -> Bus Creator9/3  "prop CL* 3"
  Demux7/4 -> Bus Creator9/4  "prop CL* 4"
  Select rows1/7 -> Demux7/1
  Bus Creator9/1 -> Bus Creator12/1  "Propeller CL*"
  Select rows1/8 -> Demux6/1
  Demux6/7 -> Bus Creator8/7  "prop CDi* 7"
  Demux6/8 -> Bus Creator8/8  "prop CDi* 8"
  Demux6/6 -> Bus Creator8/6  "prop CDi* 6"
  Demux6/5 -> Bus Creator8/5  "prop CDi* 5"
  Demux6/1 -> Bus Creator8/1  "prop CDi* 1"
  Demux6/2 -> Bus Creator8/2  "prop CDi* 2"
  Demux6/3 -> Bus Creator8/3  "prop CDi* 3"
  Demux6/4 -> Bus Creator8/4  "prop CDi* 4"
  Bus Creator11/1 -> Empennage/1  "Empennage"
  Bus Creator12/1 -> Propeller/1  "Propeller"

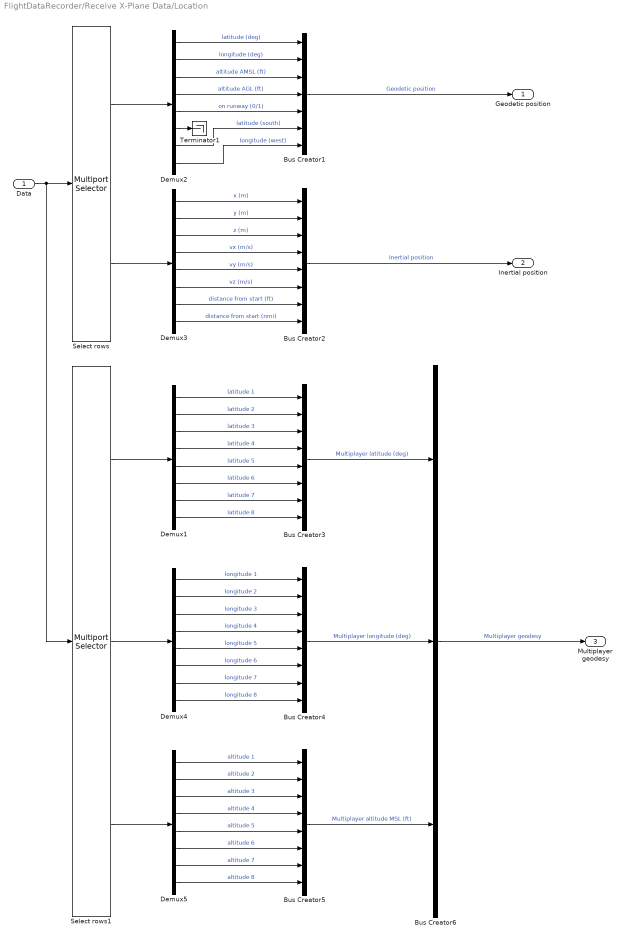
== system FlightDataRecorder/Receive X-Plane Data/Location ==
  Data : Inport
  Bus Creator1 : BusCreator  Inputs=7
  Bus Creator{2..5} (4 alike) : BusCreator  Inputs=8
  Bus Creator6 : BusCreator  Inputs=3
  Demux{1..5} (5 alike) : Demux  Outputs=8
  Select rows : dspindex/Multiport Selector  rowsOrCols=Rows  idxCellArray={21,22}  idxErrMode=Clip Index
  Select rows1 : dspindex/Multiport Selector  rowsOrCols=Rows  idxCellArray={23,24,25}  idxErrMode=Clip Index
  Terminator1 : Terminator
  Geodetic position : Outport
  Inertial position : Outport  Port=2
  Multiplayer geodesy : Outport  Port=3
  wires:
  Demux3/8 -> Bus Creator2/8  "distance from start (nmi)"
  Demux3/7 -> Bus Creator2/7  "distance from start (ft)"
  Demux3/6 -> Bus Creator2/6  "vz (m/s)"
  Demux3/5 -> Bus Creator2/5  "vy (m/s)"
  Demux3/4 -> Bus Creator2/4  "vx (m/s)"
  Data/1 -> Select rows1/1, Select rows/1
  Select rows/1 -> Demux2/1
  Select rows/2 -> Demux3/1
  Bus Creator1/1 -> Geodetic position/1  "Geodetic position"
  Demux2/8 -> Bus Creator1/7  "longitude (west)"
  Demux2/1 -> Bus Creator1/1  "latitude (deg)"
  Demux2/2 -> Bus Creator1/2  "longitude (deg)"
  Demux2/3 -> Bus Creator1/3  "altitude AMSL (ft)"
  Demux2/4 -> Bus Creator1/4  "altitude AGL (ft)"
  Demux2/5 -> Bus Creator1/5  "on runway (0/1)"
  Demux2/6 -> Terminator1/1
  Demux2/7 -> Bus Creator1/6  "latitude (south)"
  Demux3/1 -> Bus Creator2/1  "x (m)"
  Demux3/2 -> Bus Creator2/2  "y (m)"
  Demux3/3 -> Bus Creator2/3  "z (m)"
  Bus Creator2/1 -> Inertial position/1  "Inertial position"
  Demux1/8 -> Bus Creator3/8  "latitude 8"
  Demux1/7 -> Bus Creator3/7  "latitude 7"
  Demux1/6 -> Bus Creator3/6  "latitude 6"
  Demux1/5 -> Bus Creator3/5  "latitude 5"
  Demux1/4 -> Bus Creator3/4  "latitude 4"
  Select rows1/1 -> Demux1/1
  Demux1/1 -> Bus Creator3/1  "latitude 1"
  Demux1/2 -> Bus Creator3/2  "latitude 2"
  Demux1/3 -> Bus Creator3/3  "latitude 3"
  Bus Creator3/1 -> Bus Creator6/1  "Multiplayer latitude (deg)"
  Demux4/8 -> Bus Creator4/8  "longitude 8"
  Demux4/7 -> Bus Creator4/7  "longitude 7"
  Demux4/6 -> Bus Creator4/6  "longitude 6"
  Demux4/5 -> Bus Creator4/5  "longitude 5"
  Demux4/4 -> Bus Creator4/4  "longitude 4"
  Select rows1/2 -> Demux4/1
  Demux4/1 -> Bus Creator4/1  "longitude 1"
  Demux4/2 -> Bus Creator4/2  "longitude 2"
  Demux4/3 -> Bus Creator4/3  "longitude 3"
  Bus Creator4/1 -> Bus Creator6/2  "Multiplayer longitude (deg)"
  Demux5/8 -> Bus Creator5/8  "altitude 8"
  Demux5/7 -> Bus Creator5/7  "altitude 7"
  Demux5/6 -> Bus Creator5/6  "altitude 6"
  Demux5/5 -> Bus Creator5/5  "altitude 5"
  Demux5/4 -> Bus Creator5/4  "altitude 4"
  Demux5/1 -> Bus Creator5/1  "altitude 1"
  Demux5/2 -> Bus Creator5/2  "altitude 2"
  Demux5/3 -> Bus Creator5/3  "altitude 3"
  Bus Creator5/1 -> Bus Creator6/3  "Multiplayer altitude MSL (ft)"
  Select rows1/3 -> Demux5/1
  Bus Creator6/1 -> Multiplayer geodesy/1  "Multiplayer geodesy"

== system FlightDataRecorder/Receive X-Plane Data/Performance ==
  note: sm = statute miles
      | smpg = seat miles per gallon
  Data : Inport
  Bus Creator1 : BusCreator  Inputs=2
  Bus Creator2 : BusCreator  Inputs=6
  Demux1 : Demux  Outputs=8
  Demux2 : Demux  Outputs=8
  Select rows1 : dspindex/Multiport Selector  rowsOrCols=Rows  idxCellArray={133,134}  idxErrMode=Clip Index
  Terminator{1..8} (8 alike) : Terminator
  Climb performance : Outport
  Cruise performance : Outport  Port=2
  wires:
  Bus Creator2/1 -> Cruise performance/1  "Cruise performance"
  Select rows1/2 -> Demux2/1
  Demux2/1 -> Bus Creator2/1  "fuel flow (lb/hr)"
  Demux2/2 -> Bus Creator2/2  "fuel flow (gal/hr)"
  Data/1 -> Select rows1/1
  Demux2/3 -> Terminator4/1  "Vtrue (mph)"
  Demux2/8 -> Terminator5/1  "mult"
  Demux2/6 -> Bus Creator2/5  "range (sm)"
  Demux2/4 -> Bus Creator2/3  "eta (smpg)"
  Demux2/5 -> Bus Creator2/4  "eta (nmi/lb)"
  Demux2/7 -> Bus Creator2/6  "endurance (hr)"
  Bus Creator1/1 -> Climb performance/1  "Climb performance"
  Select rows1/1 -> Demux1/1
  Demux1/1 -> Bus Creator1/1  "h-spd (kt)"
  Demux1/2 -> Bus Creator1/2  "v-spd (fpm)"
  Demux1/3 -> Terminator1/1
  Demux1/4 -> Terminator2/1  "mult"
  Demux1/5 -> Terminator3/1
  Demux1/6 -> Terminator6/1
  Demux1/7 -> Terminator7/1
  Demux1/8 -> Terminator8/1
